simulink model "subsistema_pichudo"  (Simulink 7.7)
settings: Solver=ode45  StartTime=0.0  StopTime=50  RelTol=1e-3
undefined symbols (not defined in the file or in its folder): Ts
settings Model: Creator=George  LastModifiedBy=George

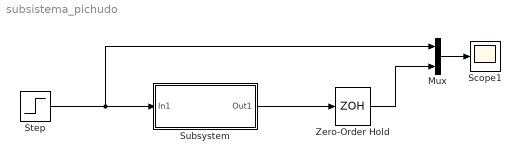
== system subsistema_pichudo ==
  Mux : Mux  Inputs=2
  Scope1 : Scope
      settings: TimeRange=20  YMin=0.3  YMax=0.7000000000000002  DataFormat=Structure  MaxDataPoints=250  SampleInput=on  SampleTime=0.02
  Step : Step  After=5  SampleTime=0.01
  Subsystem : Subsystem
  Zero-Order Hold : ZeroOrderHold  SampleTime=Ts
  wires:
  Subsystem/1(Out1) -> Zero-Order Hold/1
  Mux/1 -> Scope1/1
  Step/1 -> Subsystem/1(In1), Mux/1
  Zero-Order Hold/1 -> Mux/2

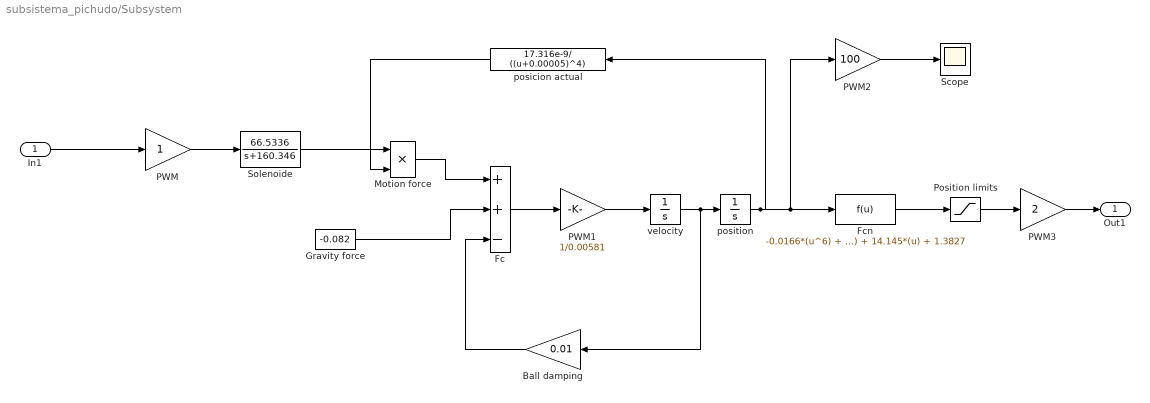
== system subsistema_pichudo/Subsystem ==
  In1 : Inport
  Ball damping : Gain  Gain=0.01  SaturateOnIntegerOverflow=on  OutDataTypeStr=Inherit: Same as input  ParamDataTypeStr=Inherit: Same as input
  Fc : Sum  Inputs=++-  SaturateOnIntegerOverflow=on  InputSameDT=on  OutDataTypeStr=Inherit: Same as first input
  Fcn : Fcn  Expr=-0.0166*(u^6) + 0.3252*(u^5) - 2.5048*(u^4) + 9.507*(u^3) - 17.977*(u^2) + 14.145*(u) + 1.3827
  Gravity force : Constant  Value=-0.082
  Motion force : Product  SaturateOnIntegerOverflow=on  InputSameDT=on  OutDataTypeStr=Inherit: Same as first input
  PWM : Gain  SaturateOnIntegerOverflow=on  OutDataTypeStr=Inherit: Same as input  ParamDataTypeStr=Inherit: Same as input
  PWM1 : Gain  Gain=1/0.00581  SaturateOnIntegerOverflow=on  OutDataTypeStr=Inherit: Same as input  ParamDataTypeStr=Inherit: Same as input
  PWM2 : Gain  Gain=100  SaturateOnIntegerOverflow=on  OutDataTypeStr=Inherit: Same as input  ParamDataTypeStr=Inherit: Same as input
  PWM3 : Gain  Gain=2  SaturateOnIntegerOverflow=on  OutDataTypeStr=Inherit: Same as input  ParamDataTypeStr=Inherit: Same as input
  Position limits : Saturate  UpperLimit=5  LowerLimit=-5  ZeroCross=off
  Scope : Scope
  Solenoide : TransferFcn  Numerator=[66.5336]  Denominator=[1 160.346]
  posicion actual : Fcn  Expr=17.316e-9/ ((u+0.00005)^4)
  position : Integrator  LimitOutput=on  UpperSaturationLimit=0.06  LowerSaturationLimit=0  ZeroCross=off
  velocity : Integrator  UpperSaturationLimit=Inf  LowerSaturationLimit=-Inf  ZeroCross=off
  Out1 : Outport
  wires:
  PWM/1 -> Solenoide/1
  Solenoide/1 -> Motion force/1
  Gravity force/1 -> Fc/2
  Motion force/1 -> Fc/1
  velocity/1 -> position/1, Ball damping/1
  position/1 -> posicion actual/1, Fcn/1, PWM2/1
  Ball damping/1 -> Fc/3
  posicion actual/1 -> Motion force/2
  Fcn/1 -> Position limits/1
  In1/1 -> PWM/1
  PWM1/1 -> velocity/1
  Fc/1 -> PWM1/1
  PWM2/1 -> Scope/1
  Position limits/1 -> PWM3/1
  PWM3/1 -> Out1/1
